simulink model "examplepressuredrop"  (Simulink 7.6)
settings: Solver=ode45  StartTime=0.0  StopTime=100  RelTol=1e-3
libraries: lib_Pressuredrop x1, simulink x1
settings Model: Creator=drhf  LastModifiedBy=drhf

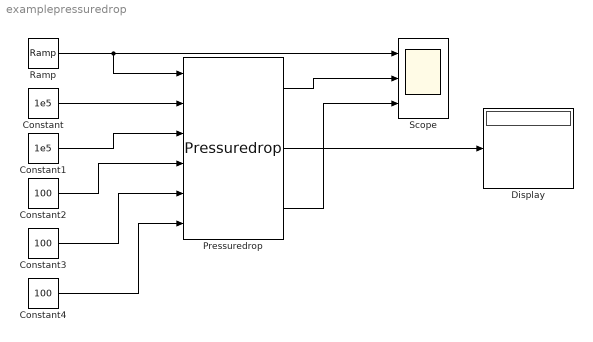
== system examplepressuredrop ==
  Constant : Constant  Value=1e5
  Constant1 : Constant  Value=1e5
  Constant2 : Constant  Value=100
  Constant3 : Constant  Value=100
  Constant4 : Constant  Value=100
  Display : Display
  Pressuredrop : lib_Pressuredrop/Pressuredrop  SystemSampleTime=-1
  Ramp : simulink/Sources/Ramp  SystemSampleTime=-1  slope=1  start=0  X0=0
  Scope : Scope  NumInputPorts=3
      settings: YMin=-5~-5~-5  YMax=5~5~5
  wires:
  Ramp/1 -> Pressuredrop/1, Scope/1
  Constant/1 -> Pressuredrop/2
  Constant1/1 -> Pressuredrop/3
  Constant2/1 -> Pressuredrop/4
  Constant3/1 -> Pressuredrop/5
  Constant4/1 -> Pressuredrop/6
  Pressuredrop/2 -> Display/1
  Pressuredrop/3 -> Scope/3
  Pressuredrop/1 -> Scope/2
